simulink model "Get_param_Ku_Tu"  (R2019a)
settings: Solver=VariableStepAuto  StartTime=0.0  StopTime=300  MaxStep=0.5  RelTol=1e-3
values from neighbouring files (symbols this model uses):
  d = 4    [parameters_D_A_Tu_Ku.m]
  plant_1 = tf([K], conv([T1,1],[T2,1]))    [plant.m]
settings Model: Creator=user1  LastModifiedBy=user1
settings SolverCC: ZeroCrossControl=DisableAll

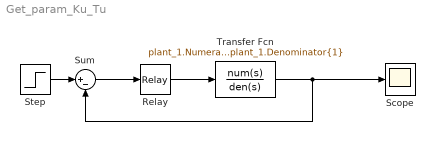
== system Get_param_Ku_Tu ==
  Relay : Relay  OnOutputValue=d  OffOutputValue=-d
  Scope : Scope
  Step : Step  Time=0  After=0  SampleTime=0
  Sum : Sum  Inputs=|+-
  Transfer Fcn : TransferFcn  Numerator=plant_1.Numerator{1}  Denominator=plant_1.Denominator{1}
  wires:
  Transfer Fcn/1 -> Sum/2, Scope/1
  Relay/1 -> Transfer Fcn/1
  Step/1 -> Sum/1
  Sum/1 -> Relay/1
